simulink model "Simulink_Control_BlueROVtest6"  (R2022b)
settings: Solver=VariableStepAuto  StartTime=0.0  StopTime=20  RelTol=1e-3
model workspace (MAT data in the model file):
  Minv : Simulink.Parameter (value not decoded)
values from neighbouring files (symbols this model uses):
  B = 0    [Control_BlueROV_Modo_Deslizante.m]
  C = 1    [Control_BlueROV_Modo_Deslizante.m]
  epsilong = 1    [Control_BlueROV_Modo_Deslizante.m]
  Ix = 0.1836    [Control_BlueROV_Modo_Deslizante.m]
  Ixy = 0    [Control_BlueROV_Modo_Deslizante.m]
  Ixz = 0    [Control_BlueROV_Modo_Deslizante.m]
  Iy = 0.2181    [Control_BlueROV_Modo_Deslizante.m]
  Iyz = -0.0021    [Control_BlueROV_Modo_Deslizante.m]
  Iz = 0.1482    [Control_BlueROV_Modo_Deslizante.m]
  K = 5    [Control_BlueROV_Modo_Deslizante.m]
  Kp = -5.005    [Control_BlueROV_Modo_Deslizante.m]
  Kpdot = -0.8576    [Control_BlueROV_Modo_Deslizante.m]
  Kpp = -80.25    [Control_BlueROV_Modo_Deslizante.m]
  m = 10.7668    [Control_BlueROV_Modo_Deslizante.m]
  M = Mrb+Ma    [Control_BlueROV_Modo_Deslizante.m]
  Minv = inv(M)    [Control_BlueROV_Modo_Deslizante.m]
  Mq = -5.005    [Control_BlueROV_Modo_Deslizante.m]
  Mqdot = -1.1214    [Control_BlueROV_Modo_Deslizante.m]
  Mqq = -80.25    [Control_BlueROV_Modo_Deslizante.m]
  Nr = -0.004    [Control_BlueROV_Modo_Deslizante.m]
  Nrdot = -0.7399    [Control_BlueROV_Modo_Deslizante.m]
  Nrr = -0.2506    [Control_BlueROV_Modo_Deslizante.m]
  W = 0    [Control_BlueROV_Modo_Deslizante.m]
  xb = 0    [Control_BlueROV_Modo_Deslizante.m]
  xg = 0    [Control_BlueROV_Modo_Deslizante.m]
  Xu = -0.0048    [Control_BlueROV_Modo_Deslizante.m]
  Xudot = -4.9063    [Control_BlueROV_Modo_Deslizante.m]
  Xuu = -30.61    [Control_BlueROV_Modo_Deslizante.m]
  yb = 0    [Control_BlueROV_Modo_Deslizante.m]
  yg = 0    [Control_BlueROV_Modo_Deslizante.m]
  Yv = -0.2437    [Control_BlueROV_Modo_Deslizante.m]
  Yvdot = -9.9210    (= -9.921)    [Control_BlueROV_Modo_Deslizante.m]
  Yvv = -38.0036    [Control_BlueROV_Modo_Deslizante.m]
  zb = 0.02    [Control_BlueROV_Modo_Deslizante.m]
  zg = 0    [Control_BlueROV_Modo_Deslizante.m]
  Zw = -0.0094    [Control_BlueROV_Modo_Deslizante.m]
  Zwdot = -17.6159    [Control_BlueROV_Modo_Deslizante.m]
  Zww = -62.5364    [Control_BlueROV_Modo_Deslizante.m]
libraries: simulink x1
(part 3 of 3)

== matlab function Simulink_Control_BlueROVtest6/Sliding Mode Control/Inv(J(n)) ==
  data: phi input; y output; theta input; psi input
function y = fcn(phi,theta,psi)

y = [((((sin(phi)*sin(psi) + sin(theta)*cos(phi)*cos(psi))*sin(theta) + cos(phi)*cos(psi)*cos(theta)^2)*((sin(phi)*sin(psi)*sin(theta) + cos(phi)*cos(psi))*cos(psi)*cos(theta) - (sin(phi)*sin(theta)*cos(psi) - sin(psi)*cos(phi))*sin(psi)*cos(theta)) - ((sin(phi)*sin(theta)*cos(psi) - sin(psi)*cos(phi))*sin(theta) + sin(phi)*cos(psi)*cos(theta)^2)*(-(sin(phi)*sin(psi) + sin(theta)*cos(phi)*cos(psi))*sin(psi)*cos(theta) + (-sin(phi)*cos(psi) + sin(psi)*sin(theta)*cos(phi))*cos(psi)*cos(theta)))*(sin(phi)*sin(psi)*sin(theta) + cos(phi)*cos(psi))*cos(psi)*cos(theta) - ((sin(phi)*sin(psi) + sin(theta)*cos(phi)*cos(psi))*((sin(phi)*sin(psi)*sin(theta) + cos(phi)*cos(psi))*cos(psi)*cos(theta) - (sin(phi)*sin(theta)*cos(psi) - sin(psi)*cos(phi))*sin(psi)*cos(theta)) - (-(sin(phi)*sin(psi) + sin(theta)*cos(phi)*cos(psi))*sin(psi)*cos(theta) + (-sin(phi)*cos(psi) + sin(psi)*sin(theta)*cos(phi))*cos(psi)*cos(theta))*(sin(phi)*sin(theta)*cos(psi) - sin(psi)*cos(phi)))*(((sin(phi)*sin(theta)*cos(psi) - sin(psi)*cos(phi))*sin(theta) + sin(phi)*cos(psi)*cos(theta)^2)*sin(psi)*cos(theta) + ((sin(phi)*sin(psi)*sin(theta) + cos(phi)*cos(psi))*cos(psi)*cos(theta) - (sin(phi)*sin(theta)*cos(psi) - sin(psi)*cos(phi))*sin(psi)*cos(theta))*sin(theta)))/((((sin(phi)*sin(psi) + sin(theta)*cos(phi)*cos(psi))*sin(theta) + cos(phi)*cos(psi)*cos(theta)^2)*((sin(phi)*sin(psi)*sin(theta) + cos(phi)*cos(psi))*cos(psi)*cos(theta) - (sin(phi)*sin(theta)*cos(psi) - sin(psi)*cos(phi))*sin(psi)*cos(theta)) - ((sin(phi)*sin(theta)*cos(psi) - sin(psi)*cos(phi))*sin(theta) + sin(phi)*cos(psi)*cos(theta)^2)*(-(sin(phi)*sin(psi) + sin(theta)*cos(phi)*cos(psi))*sin(psi)*cos(theta) + (-sin(phi)*cos(psi) + sin(psi)*sin(theta)*cos(phi))*cos(psi)*cos(theta)))*((sin(phi)*sin(psi)*sin(theta) + cos(phi)*cos(psi))*cos(psi)*cos(theta) - (sin(phi)*sin(theta)*cos(psi) - sin(psi)*cos(phi))*sin(psi)*cos(theta))*cos(psi)*cos(theta)), (-(((sin(phi)*sin(psi) + sin(theta)*cos(phi)*cos(psi))*sin(theta) + cos(phi)*cos(psi)*cos(theta)^2)*((sin(phi)*sin(psi)*sin(theta) + cos(phi)*cos(psi))*cos(psi)*cos(theta) - (sin(phi)*sin(theta)*cos(psi) - sin(psi)*cos(phi))*sin(psi)*cos(theta)) - ((sin(phi)*sin(theta)*cos(psi) - sin(psi)*cos(phi))*sin(theta) + sin(phi)*cos(psi)*cos(theta)^2)*(-(sin(phi)*sin(psi) + sin(theta)*cos(phi)*cos(psi))*sin(psi)*cos(theta) + (-sin(phi)*cos(psi) + sin(psi)*sin(theta)*cos(phi))*cos(psi)*cos(theta)))*(sin(phi)*sin(theta)*cos(psi) - sin(psi)*cos(phi))*cos(psi)*cos(theta) + ((sin(phi)*sin(psi) + sin(theta)*cos(phi)*cos(psi))*((sin(phi)*sin(psi)*sin(theta) + cos(phi)*cos(psi))*cos(psi)*cos(theta) - (sin(phi)*sin(theta)*cos(psi) - sin(psi)*cos(phi))*sin(psi)*cos(theta)) - (-(sin(phi)*sin(psi) + sin(theta)*cos(phi)*cos(psi))*sin(psi)*cos(theta) + (-sin(phi)*cos(psi) + sin(psi)*sin(theta)*cos(phi))*cos(psi)*cos(theta))*(sin(phi)*sin(theta)*cos(psi) - sin(psi)*cos(phi)))*((sin(phi)*sin(theta)*cos(psi) - sin(psi)*cos(phi))*sin(theta) + sin(phi)*cos(psi)*cos(theta)^2)*cos(psi)*cos(theta))/((((sin(phi)*sin(psi) + sin(theta)*cos(phi)*cos(psi))*sin(theta) + cos(phi)*cos(psi)*cos(theta)^2)*((sin(phi)*sin(psi)*sin(theta) + cos(phi)*cos(psi))*cos(psi)*cos(theta) - (sin(phi)*sin(theta)*cos(psi) - sin(psi)*cos(phi))*sin(psi)*cos(theta)) - ((sin(phi)*sin(theta)*cos(psi) - sin(psi)*cos(phi))*sin(theta) + sin(phi)*cos(psi)*cos(theta)^2)*(-(sin(phi)*sin(psi) + sin(theta)*cos(phi)*cos(psi))*sin(psi)*cos(theta) + (-sin(phi)*cos(psi) + sin(psi)*sin(theta)*cos(phi))*cos(psi)*cos(theta)))*((sin(phi)*sin(psi)*sin(theta) + cos(phi)*cos(psi))*cos(psi)*cos(theta) - (sin(phi)*sin(theta)*cos(psi) - sin(psi)*cos(phi))*sin(psi)*cos(theta))*cos(psi)*cos(theta)), -((sin(phi)*sin(psi) + sin(theta)*cos(phi)*cos(psi))*((sin(phi)*sin(psi)*sin(theta) + cos(phi)*cos(psi))*cos(psi)*cos(theta) - (sin(phi)*sin(theta)*cos(psi) - sin(psi)*cos(phi))*sin(psi)*cos(theta)) - (-(sin(phi)*sin(psi) + sin(theta)*cos(phi)*cos(psi))*sin(psi)*cos(theta) + (-sin(phi)*cos(psi) + sin(psi)*sin(theta)*cos(phi))*cos(psi)*cos(theta))*(sin(phi)*sin(theta)*cos(psi) - sin(psi)*cos(phi)))/(((sin(phi)*sin(psi) + sin(theta)*cos(phi)*cos(psi))*sin(theta) + cos(phi)*cos(psi)*cos(theta)^2)*((sin(phi)*sin(psi)*sin(theta) + cos(phi)*cos(psi))*cos(psi)*cos(theta) - (sin(phi)*sin(theta)*cos(psi) - sin(psi)*cos(phi))*sin(psi)*cos(theta)) - ((sin(phi)*sin(theta)*cos(psi) - sin(psi)*cos(phi))*sin(theta) + sin(phi)*cos(psi)*cos(theta)^2)*(-(sin(phi)*sin(psi) + sin(theta)*cos(phi)*cos(psi))*sin(psi)*cos(theta) + (-sin(phi)*cos(psi) + sin(psi)*sin(theta)*cos(phi))*cos(psi)*cos(theta))), 0, 0, 0;(-(((sin(phi)*sin(psi) + sin(theta)*cos(phi)*cos(psi))*sin(theta) + cos(phi)*cos(psi)*cos(theta)^2)*((sin(phi)*sin(psi)*sin(theta) + cos(phi)*cos(psi))*cos(psi)*cos(theta) - (sin(phi)*sin(theta)*cos(psi) - sin(psi)*cos(phi))*sin(psi)*cos(theta)) - ((sin(phi)*sin(theta)*cos(psi) - sin(psi)*cos(phi))*sin(theta) + sin(phi)*cos(psi)*cos(theta)^2)*(-(sin(phi)*sin(psi) + sin(theta)*cos(phi)*cos(psi))*sin(psi)*cos(theta) + (-sin(phi)*cos(psi) + sin(psi)*sin(theta)*cos(phi))*cos(psi)*cos(theta)))*sin(psi)*cos(theta) - (((sin(phi)*sin(theta)*cos(psi) - sin(psi)*cos(phi))*sin(theta) + sin(phi)*cos(psi)*cos(theta)^2)*sin(psi)*cos(theta) + ((sin(phi)*sin(psi)*sin(theta) + cos(phi)*cos(psi))*cos(psi)*cos(theta) - (sin(phi)*sin(theta)*cos(psi) - sin(psi)*cos(phi))*sin(psi)*cos(theta))*sin(theta))*(-(sin(phi)*sin(psi) + sin(theta)*cos(phi)*cos(psi))*sin(psi)*cos(theta) + (-sin(phi)*cos(psi) + sin(psi)*sin(theta)*cos(phi))*cos(psi)*cos(theta)))/((((sin(phi)*sin(psi) + sin(theta)*cos(phi)*cos(psi))*sin(theta) + cos(phi)*cos(psi)*cos(theta)^2)*((sin(phi)*sin(psi)*sin(theta) + cos(phi)*cos(psi))*cos(psi)*cos(theta) - (sin(phi)*sin(theta)*cos(psi) - sin(psi)*cos(phi))*sin(psi)*cos(theta)) - ((sin(phi)*sin(theta)*cos(psi) - sin(psi)*cos(phi))*sin(theta) + sin(phi)*cos(psi)*cos(theta)^2)*(-(sin(phi)*sin(psi) + sin(theta)*cos(phi)*cos(psi))*sin(psi)*cos(theta) + (-sin(phi)*cos(psi) + sin(psi)*sin(theta)*cos(phi))*cos(psi)*cos(theta)))*((sin(phi)*sin(psi)*sin(theta) + cos(phi)*cos(psi))*cos(psi)*cos(theta) - (sin(phi)*sin(theta)*cos(psi) - sin(psi)*cos(phi))*sin(psi)*cos(theta))), ((((sin(phi)*sin(psi) + sin(theta)*cos(phi)*cos(psi))*sin(theta) + cos(phi)*cos(psi)*cos(theta)^2)*((sin(phi)*sin(psi)*sin(theta) + cos(phi)*cos(psi))*cos(psi)*cos(theta) - (sin(phi)*sin(theta)*cos(psi) - sin(psi)*cos(phi))*sin(psi)*cos(theta)) - ((sin(phi)*sin(theta)*cos(psi) - sin(psi)*cos(phi))*sin(theta) + sin(phi)*cos(psi)*cos(theta)^2)*(-(sin(phi)*sin(psi) + sin(theta)*cos(phi)*cos(psi))*sin(psi)*cos(theta) + (-sin(phi)*cos(psi) + sin(psi)*sin(theta)*cos(phi))*cos(psi)*cos(theta)))*cos(psi)*cos(theta) + ((sin(phi)*sin(theta)*cos(psi) - sin(psi)*cos(phi))*sin(theta) + sin(phi)*cos(psi)*cos(theta)^2)*(-(sin(phi)*sin(psi) + sin(theta)*cos(phi)*cos(psi))*sin(psi)*cos(theta) + (-sin(phi)*cos(psi) + sin(psi)*sin(theta)*cos(phi))*cos(psi)*cos(theta))*cos(psi)*cos(theta))/((((sin(phi)*sin(psi) + sin(theta)*cos(phi)*cos(psi))*sin(theta) + cos(phi)*cos(psi)*cos(theta)^2)*((sin(phi)*sin(psi)*sin(theta) + cos(phi)*cos(psi))*cos(psi)*cos(theta) - (sin(phi)*sin(theta)*cos(psi) - sin(psi)*cos(phi))*sin(psi)*cos(theta)) - ((sin(phi)*sin(theta)*cos(psi) - sin(psi)*cos(phi))*sin(theta) + sin(phi)*cos(psi)*cos(theta)^2)*(-(sin(phi)*sin(psi) + sin(theta)*cos(phi)*cos(psi))*sin(psi)*cos(theta) + (-sin(phi)*cos(psi) + sin(psi)*sin(theta)*cos(phi))*cos(psi)*cos(theta)))*((sin(phi)*sin(psi)*sin(theta) + cos(phi)*cos(psi))*cos(psi)*cos(theta) - (sin(phi)*sin(theta)*cos(psi) - sin(psi)*cos(phi))*sin(psi)*cos(theta))), -(-(sin(phi)*sin(psi) + sin(theta)*cos(phi)*cos(psi))*sin(psi)*cos(theta) + (-sin(phi)*cos(psi) + sin(psi)*sin(theta)*cos(phi))*cos(psi)*cos(theta))*cos(psi)*cos(theta)/(((sin(phi)*sin(psi) + sin(theta)*cos(phi)*cos(psi))*sin(theta) + cos(phi)*cos(psi)*cos(theta)^2)*((sin(phi)*sin(psi)*sin(theta) + cos(phi)*cos(psi))*cos(psi)*cos(theta) - (sin(phi)*sin(theta)*cos(psi) - sin(psi)*cos(phi))*sin(psi)*cos(theta)) - ((sin(phi)*sin(theta)*cos(psi) - sin(psi)*cos(phi))*sin(theta) + sin(phi)*cos(psi)*cos(theta)^2)*(-(sin(phi)*sin(psi) + sin(theta)*cos(phi)*cos(psi))*sin(psi)*cos(theta) + (-sin(phi)*cos(psi) + sin(psi)*sin(theta)*cos(phi))*cos(psi)*cos(theta))), 0, 0, 0;(((sin(phi)*sin(theta)*cos(psi) - sin(psi)*cos(phi))*sin(theta) + sin(phi)*cos(psi)*cos(theta)^2)*sin(psi)*cos(theta) + ((sin(phi)*sin(psi)*sin(theta) + cos(phi)*cos(psi))*cos(psi)*cos(theta) - (sin(phi)*sin(theta)*cos(psi) - sin(psi)*cos(phi))*sin(psi)*cos(theta))*sin(theta))/(((sin(phi)*sin(psi) + sin(theta)*cos(phi)*cos(psi))*sin(theta) + cos(phi)*cos(psi)*cos(theta)^2)*((sin(phi)*sin(psi)*sin(theta) + cos(phi)*cos(psi))*cos(psi)*cos(theta) - (sin(phi)*sin(theta)*cos(psi) - sin(psi)*cos(phi))*sin(psi)*cos(theta)) - ((sin(phi)*sin(theta)*cos(psi) - sin(psi)*cos(phi))*sin(theta) + sin(phi)*cos(psi)*cos(theta)^2)*(-(sin(phi)*sin(psi) + sin(theta)*cos(phi)*cos(psi))*sin(psi)*cos(theta) + (-sin(phi)*cos(psi) + sin(psi)*sin(theta)*cos(phi))*cos(psi)*cos(theta))), -((sin(phi)*sin(theta)*cos(psi) - sin(psi)*cos(phi))*sin(theta) + sin(phi)*cos(psi)*cos(theta)^2)*cos(psi)*cos(theta)/(((sin(phi)*sin(psi) + sin(theta)*cos(phi)*cos(psi))*sin(theta) + cos(phi)*cos(psi)*cos(theta)^2)*((sin(phi)*sin(psi)*sin(theta) + cos(phi)*cos(psi))*cos(psi)*cos(theta) - (sin(phi)*sin(theta)*cos(psi) - sin(psi)*cos(phi))*sin(psi)*cos(theta)) - ((sin(phi)*sin(theta)*cos(psi) - sin(psi)*cos(phi))*sin(theta) + sin(phi)*cos(psi)*cos(theta)^2)*(-(sin(phi)*sin(psi) + sin(theta)*cos(phi)*cos(psi))*sin(psi)*cos(theta) + (-sin(phi)*cos(psi) + sin(psi)*sin(theta)*cos(phi))*cos(psi)*cos(theta))), ((sin(phi)*sin(psi)*sin(theta) + cos(phi)*cos(psi))*cos(psi)*cos(theta) - (sin(phi)*sin(theta)*cos(psi) - sin(psi)*cos(phi))*sin(psi)*cos(theta))*cos(psi)*cos(theta)/(((sin(phi)*sin(psi) + sin(theta)*cos(phi)*cos(psi))*sin(theta) + cos(phi)*cos(psi)*cos(theta)^2)*((sin(phi)*sin(psi)*sin(theta) + cos(phi)*cos(psi))*cos(psi)*cos(theta) - (sin(phi)*sin(theta)*cos(psi) - sin(psi)*cos(phi))*sin(psi)*cos(theta)) - ((sin(phi)*sin(theta)*cos(psi) - sin(psi)*cos(phi))*sin(theta) + sin(phi)*cos(psi)*cos(theta)^2)*(-(sin(phi)*sin(psi) + sin(theta)*cos(phi)*cos(psi))*sin(psi)*cos(theta) + (-sin(phi)*cos(psi) + sin(psi)*sin(theta)*cos(phi))*cos(psi)*cos(theta))), 0, 0, 0;0, 0, 0, 1, (-(sin(phi)^2/cos(theta) + cos(phi)^2/cos(theta))*sin(phi)*sin(theta)/cos(theta) + (sin(phi)^2*sin(theta)/cos(theta) + sin(theta)*cos(phi)^2/cos(theta))*sin(phi)/cos(theta))/((sin(phi)^2/cos(theta) + cos(phi)^2/cos(theta))*cos(phi)), -(sin(phi)^2*sin(theta)/cos(theta) + sin(theta)*cos(phi)^2/cos(theta))/(sin(phi)^2/cos(theta) + cos(phi)^2/cos(theta));0, 0, 0, 0, cos(phi)/((sin(phi)^2/cos(theta) + cos(phi)^2/cos(theta))*cos(theta)), sin(phi)/(sin(phi)^2/cos(theta) + cos(phi)^2/cos(theta));0, 0, 0, 0, -sin(phi)/((sin(phi)^2/cos(theta) + cos(phi)^2/cos(theta))*cos(theta)), cos(phi)/(sin(phi)^2/cos(theta) + cos(phi)^2/cos(theta))];

== matlab function Simulink_Control_BlueROVtest6/Sliding Mode Control/MATLAB Function1 ==
  data: B input; X_dot output; A input; T input; t input
function X_dot = fcn(B,A,T,t)

X_dot = -(2*pi/T)*(2*pi/T)*A*sin((2*pi/T)*t);

== matlab function Simulink_Control_BlueROVtest6/Sliding Mode Control/MATLAB Function4 ==
  data: s input; sgn output
function sgn = fcn(s)

    sgn=sign(s);

== matlab function Simulink_Control_BlueROVtest6/BlueRov2Heavy/MATLAB Function ==
  data: B input; x_dur output; A input; T input; t input
function x_dur = fcn(B,A,T,t)

x_dur=B+A*sin((2*pi/T)*t);

== matlab function Simulink_Control_BlueROVtest6/Sliding Mode Control/J_dot ==
  data: phi input; J_dot output; theta input; psi input; phi_dot input; theta_dot input; psi_dot input
function J_dot = fcn(phi,theta,psi,phi_dot,theta_dot,psi_dot)
% Rotation matrix to map the Euler Angle attitudes
n_1 = [1 sin(phi)*tan(theta) cos(phi)*tan(theta);
       0    cos(phi)            -sin(phi);
       0 sin(phi)*sec(theta)    cos(phi)*sec(theta)];

%Rotation matrix to map the translational velocities in the body frame
n_2 = [cos(psi)*cos(theta)    (-sin(psi)*cos(phi) + cos(psi)*sin(theta)*sin(phi)) (sin(psi)*sin(phi) + cos(psi)*cos(phi)*sin(theta));
     sin(psi)*cos(theta)    (cos(psi)*cos(phi) + sin(phi)*sin(theta)*sin(psi))  (-cos(psi)*sin(phi) + sin(theta)*sin(psi)*cos(phi));
     -sin(theta)            cos(theta)*sin(phi)                                 cos(theta)*cos(phi)];



J1_dot=[- psi_dot*cos(theta)*sin(psi) - theta_dot*cos(psi)*sin(theta), phi_dot*sin(phi)*sin(psi) - psi_dot*cos(phi)*cos(psi) + phi_dot*cos(phi)*cos(psi)*sin(theta) + theta_dot*cos(psi)*cos(theta)*sin(phi) - psi_dot*sin(phi)*sin(psi)*sin(theta), phi_dot*cos(phi)*sin(psi) + psi_dot*cos(psi)*sin(phi) + theta_dot*cos(phi)*cos(psi)*cos(theta) - phi_dot*cos(psi)*sin(phi)*sin(theta) - psi_dot*cos(phi)*sin(psi)*sin(theta); 
   psi_dot*cos(psi)*cos(theta) - theta_dot*sin(psi)*sin(theta), phi_dot*cos(phi)*sin(psi)*sin(theta) - psi_dot*cos(phi)*sin(psi) - phi_dot*cos(psi)*sin(phi) + psi_dot*cos(psi)*sin(phi)*sin(theta) + theta_dot*cos(theta)*sin(phi)*sin(psi), psi_dot*sin(phi)*sin(psi) - phi_dot*cos(phi)*cos(psi) + psi_dot*cos(phi)*cos(psi)*sin(theta) + theta_dot*cos(phi)*cos(theta)*sin(psi) - phi_dot*sin(phi)*sin(psi)*sin(theta);
 -theta_dot*cos(theta), phi_dot*cos(phi)*cos(theta) - theta_dot*sin(phi)*sin(theta), - phi_dot*cos(theta)*sin(phi) - theta_dot*cos(phi)*sin(theta)];

J2_dot=[0        phi_dot*cos(phi)*tan(theta)+sin(phi)*((tan(theta)^2)+1)*theta_dot                                        -sin(phi)*phi_dot*tan(theta)+cos(phi)*(tan(theta)^2 + 1)*theta_dot; 
              0                                              -sin(phi)*phi_dot                                                                                                                            -cos(phi)*phi_dot;
              0        cos(phi)*phi_dot*sec(theta)+sin(phi)*sin(phi)*sin(theta)/(cos(theta)^2)*theta_dot                -sin(phi)*phi_dot*sec(theta)+cos(phi)*(cos(phi)*sin(theta))/cos(theta)^2*theta_dot];
J_dot=[J1_dot  zeros(3);
              zeros(3)  J2_dot];

== matlab function Simulink_Control_BlueROVtest6/Sliding Mode Control/MATLAB Function2 ==
  data: s input; sat output
function sat = fcn(s)

delta=0.05;
k=1/delta;
if abs(s)<=delta
    sat=k*s;
else
    sat=sign(s);
end

== matlab function Simulink_Control_BlueROVtest6/Sliding Mode Control/MATLAB Function ==
  data: fL input; fc output; fU input; s input
function fc = fcn(fL,fU,s)

d1=(fU-fL)/2;
d2=(fU+fL)/2;

fc=d2+d1*sign(s);

== matlab function Simulink_Control_BlueROVtest6/Sliding Mode Control/MATLAB Function3 ==
  data: B input; X_dot output; A input; T input; t input
function X_dot = fcn(B,A,T,t)

X_dot = (2*pi/T)*A*cos((2*pi/T)*t);

== matlab function Simulink_Control_BlueROVtest6/MATLAB Function2 ==
  data: B input; SetX output; A input; T input; t input
function SetX = fcn(B,A,T,t)

SetX = B+A*sin((2*pi/T)*t);
